simulink model "HW3_virtual_testbed_3"  (R2023b)
settings: Solver=FixedStepAuto  StartTime=0.0  StopTime=Tspan  FixedStep=Delta_t  RelTol=1e-3
values from neighbouring files (symbols this model uses):
  Q = 5    [HW3.m]
undefined symbols (not defined in the file or in its folder): C1, DiscIntNeverNeededParam, OCV_Poly, R1, Rs, Soc_Init
settings Model: Creator=Spencer  LastModifiedBy=Spencer
settings DebuggingCC: AlgebraicLoopMsg=none

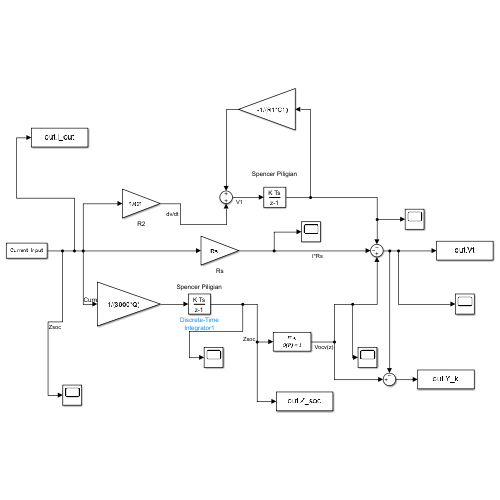
[thumbnail: Simulink's stored preview of the top-level diagram]
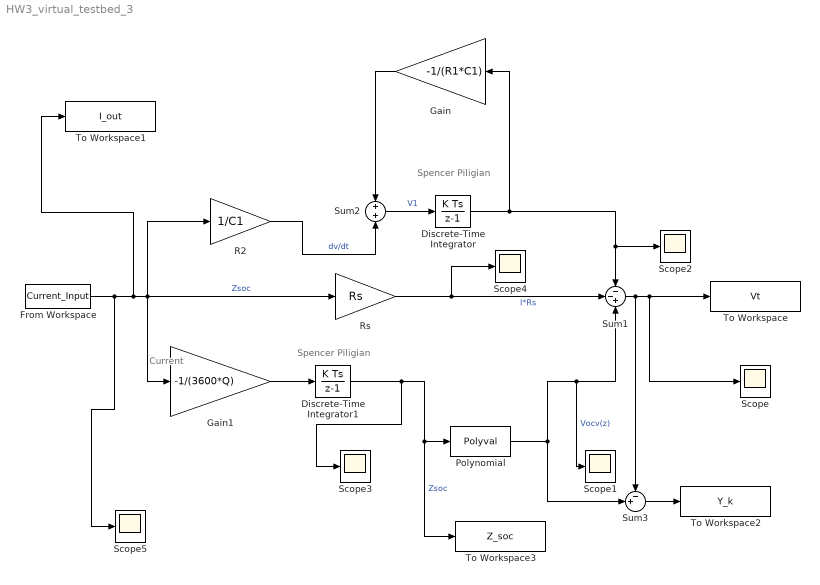
== system HW3_virtual_testbed_3 ==
  note: Spencer Piligian
  note: Current
  note: Spencer Piligian
  Discrete-Time Integrator : DiscreteIntegrator  SampleTime=-1  ICPrevOutput=DiscIntNeverNeededParam  ICPrevScaledInput=DiscIntNeverNeededParam
  Discrete-Time Integrator1 : DiscreteIntegrator  InitialCondition=Soc_Init  SampleTime=-1  ICPrevOutput=DiscIntNeverNeededParam  ICPrevScaledInput=DiscIntNeverNeededParam
  From Workspace : FromWorkspace  VariableName=Current_Input
  Gain : Gain  Gain=-1/(R1*C1)
  Gain1 : Gain  Gain=-1/(3600*Q)
  Polynomial : Polyval  Coefs=OCV_Poly
  R2 : Gain  Gain=1/C1
  Rs : Gain  Gain=Rs
  Scope{,1..5} (6 alike) : Scope
  Sum1 : Sum  Inputs=--+
  Sum2 : Sum
  Sum3 : Sum  Inputs=-+|
  To Workspace : ToWorkspace  VariableName=Vt  SampleTime=-1
      settings: Save2DSignal=2-D array (concatenate along first dimension)
  To Workspace1 : ToWorkspace  VariableName=I_out  SampleTime=-1
      settings: Save2DSignal=2-D array (concatenate along first dimension)
  To Workspace2 : ToWorkspace  VariableName=Y_k  SampleTime=-1
      settings: Save2DSignal=2-D array (concatenate along first dimension)
  To Workspace3 : ToWorkspace  VariableName=Z_soc  SampleTime=-1
      settings: Save2DSignal=2-D array (concatenate along first dimension)
  wires:
  Sum1/1 -> To Workspace/1, Scope/1, Sum3/1
  Gain1/1 -> Discrete-Time Integrator1/1
  Discrete-Time Integrator1/1 -> Scope3/1, Polynomial/1, To Workspace3/1  "Zsoc"
  Polynomial/1 -> Sum1/3, Scope1/1, Sum3/2  "Vocv(z)"
  Rs/1 -> Scope4/1, Sum1/2  "I*Rs"
  Sum2/1 -> Discrete-Time Integrator/1  "V1"
  R2/1 -> Sum2/2  "dv/dt"
  Sum3/1 -> To Workspace2/1
  Discrete-Time Integrator/1 -> Gain/1, Scope2/1, Sum1/1
  Gain/1 -> Sum2/1
  From Workspace/1 -> Scope5/1, To Workspace1/1, Rs/1, R2/1, Gain1/1  "Zsoc"
